simulink model "SensorlessBLDCMotorSimulation1"  (R2023a)
settings: Solver=VariableStepAuto  StartTime=0.0  StopTime=10.0  RelTol=1e-3
libraries: spsMosfetLib x6, spsPermanentMagnetSynchronousMachineLib x1, spsDCVoltageSourceLib x1, sps_lib x1
settings Model: Creator=ABRA A5 V16.6.1  LastModifiedBy=ABRA A5 V16.6.1

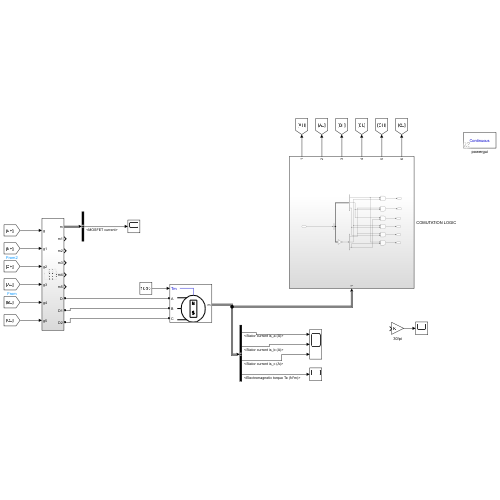
[thumbnail: Simulink's stored preview of the top-level diagram]
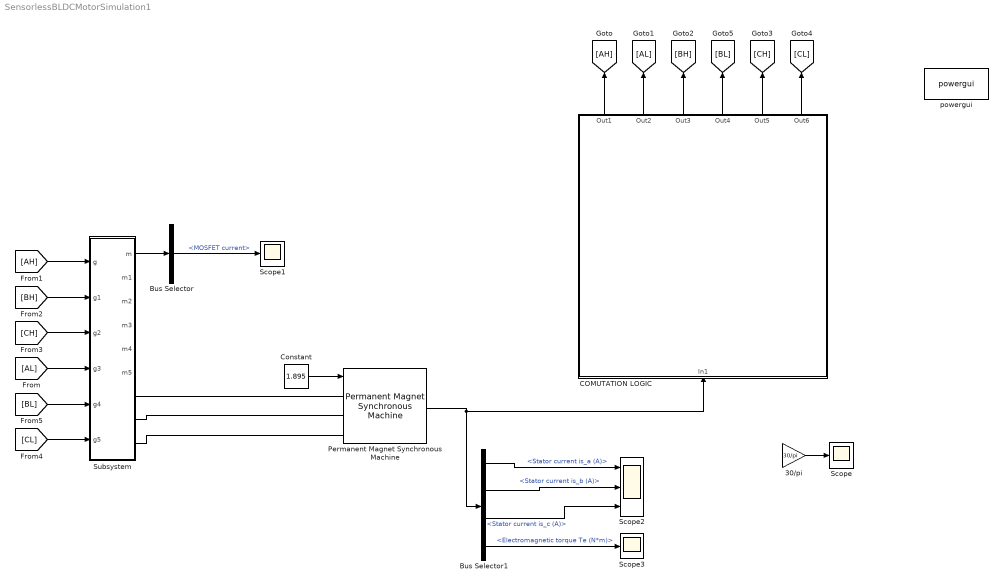
== system SensorlessBLDCMotorSimulation1 ==
  30/pi : Gain  Gain=30/pi
  Bus Selector : BusSelector  OutputSignals=MOSFET current
  Bus Selector1 : BusSelector  OutputSignals=Stator current is_a (A),Stator current is_b (A),Stator current is_c (A),Electromagnetic torque Te (N*m)
  COMUTATION LOGIC : Subsystem
  Constant : Constant  Value=1.895
  Permanent Magnet Synchronous Machine : spsPermanentMagnetSynchronousMachineLib/Permanent Magnet Synchronous Machine  NbPhases=3  FluxDistribution=Trapezoidal  RotorType=Round  MechanicalLoad=Torque Tm  PresetModel=No  ShowDetailedParameters=on  MeasurementBus=off  Resistance=0.0801  Inductance=0.0000841  dqInductances=[8.5e-3,8.5e-3]  La=0.000395  MachineConstant=Flux linkage established by magnets (V.s)  Flux=0.00216  VoltageCst=6.3335  TorqueCst=0.06048  Flat=120  Mechanical=[0.0002125 0.0004924 14 0]  PolePairs=4  InitialConditions=[314.159,-3.21, 30,30]  InitialConditions5ph=[0 0 0 0 0 0]  RefAngle=90 degrees behind phase A axis (modified Park)  IterativeDiscreteModel=Trapezoidal non iterative  TsBlock=-1  TsPowergui=0
  Scope : Scope
  Scope1 : Scope
  Scope2 : Scope  NumInputPorts=3
  Scope3 : Scope
  Subsystem : Subsystem
  powergui : sps_lib/powergui  Priority=1  SimulationMode=Continuous  SampleTime=50e-6  frequency=60  Iterations=50  frequencyindice=0  Pbase=100e6  ErrMax=1e-4  UnitsV=kV  UnitsW=MW  buscounter=0  FunctionMessages=off  echomessages=off  EnableUseOfTLC=off  CurrentSourceSwitches=off  DisableSnubberDevices=off  DisableRonSwitches=off  DisableVfSwitches=off  DisplayEquations=off  AutomaticDiscreteSolvers=off  SolverType=Tustin/Backward Euler (TBE)  Interpol=off  ExternalGateDelay=off  methode=off  Ts=100  x0status=blocks  SPID=on  SwTol=0  HookPort=off  NonlinearTolerance=1e-4  nMaxIteration=100  ContinueOnMaxIteration=off  RestoreLinks=warning  ResistiveCurrentMeasurement=off  Frange=[0:2:500]  Ylog=off  Xlog=on  ShowGrid=off  save=off  variable=ZData  structure=0  ZoomFFT=off  StartTime=0.0  cycles=1  DisplayStyle=1  fundamental=60  FreqAxis=off  MaxFrequency=1000  frequencyindicesteady=1  RmsSteady=1  display=off
  wires:
  Permanent Magnet Synchronous Machine/1 -> Bus Selector1/1, COMUTATION LOGIC/1(In1)
  COMUTATION LOGIC/1(Out1) -> [AH]
  COMUTATION LOGIC/2(Out2) -> [AL]
  COMUTATION LOGIC/3(Out3) -> [BH]
  COMUTATION LOGIC/4(Out4) -> [BL]
  COMUTATION LOGIC/5(Out5) -> [CH]
  COMUTATION LOGIC/6(Out6) -> [CL]
  [AH] -> Subsystem/1(g)
  [BH] -> Subsystem/2(g1)
  [CH] -> Subsystem/3(g2)
  [AL] -> Subsystem/4(g3)
  [BL] -> Subsystem/5(g4)
  [CL] -> Subsystem/6(g5)
  Subsystem/1(m) -> Bus Selector/1
  Bus Selector/1 -> Scope1/1  "<MOSFET current>"
  Constant/1 -> Permanent Magnet Synchronous Machine/1
  30/pi/1 -> Scope/1
  Bus Selector1/1 -> Scope2/1  "<Stator current is_a (A)>"
  Bus Selector1/2 -> Scope2/2  "<Stator current is_b (A)>"
  Bus Selector1/3 -> Scope2/3  "<Stator current is_c (A)>"
  Bus Selector1/4 -> Scope3/1  "<Electromagnetic torque Te (N*m)>"
  connections:
  Permanent Magnet Synchronous Machine/LConn1 -- Subsystem/RConn1
  Permanent Magnet Synchronous Machine/LConn2 -- Subsystem/RConn2
  Permanent Magnet Synchronous Machine/LConn3 -- Subsystem/RConn3

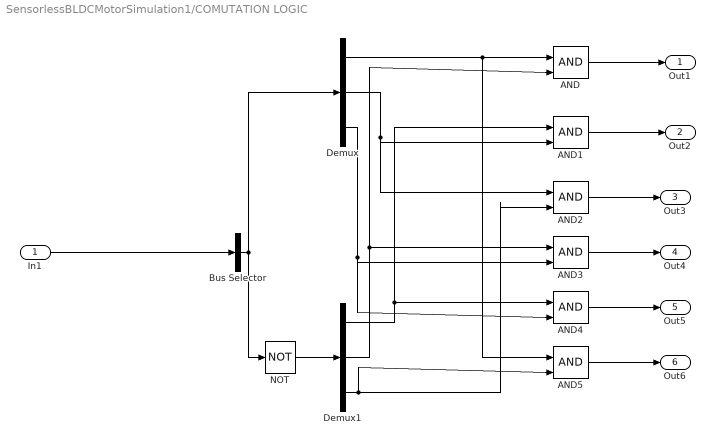
== system SensorlessBLDCMotorSimulation1/COMUTATION LOGIC ==
  In1 : Inport
  AND{,1..5} (6 alike) : Logic  IconShape=distinctive  AllPortsSameDT=off  OutDataTypeStr=boolean
  Bus Selector : BusSelector  OutputSignals=Hall effect signal h_a,Hall effect signal h_b,Hall effect signal h_c  OutputAsBus=on
  Demux : Demux  Outputs=3
  Demux1 : Demux  Outputs=3
  NOT : Logic  Operator=NOT  IconShape=distinctive  AllPortsSameDT=off  OutDataTypeStr=boolean
  Out1 : Outport
  Out2 : Outport  Port=2
  Out3 : Outport  Port=3
  Out4 : Outport  Port=4
  Out5 : Outport  Port=5
  Out6 : Outport  Port=6
  wires:
  AND3/1 -> Out4/1
  In1/1 -> Bus Selector/1
  Demux1/2 -> AND3/1, AND/2
  Bus Selector/1 -> Demux/1, NOT/1
  Demux/1 -> AND5/1, AND/1
  Demux/2 -> AND2/1, AND1/2
  Demux1/1 -> AND4/1, AND1/1
  AND4/1 -> Out5/1
  Demux1/3 -> AND5/2, AND2/2
  Demux/3 -> AND4/2, AND3/2
  AND2/1 -> Out3/1
  NOT/1 -> Demux1/1
  AND5/1 -> Out6/1
  AND/1 -> Out1/1
  AND1/1 -> Out2/1

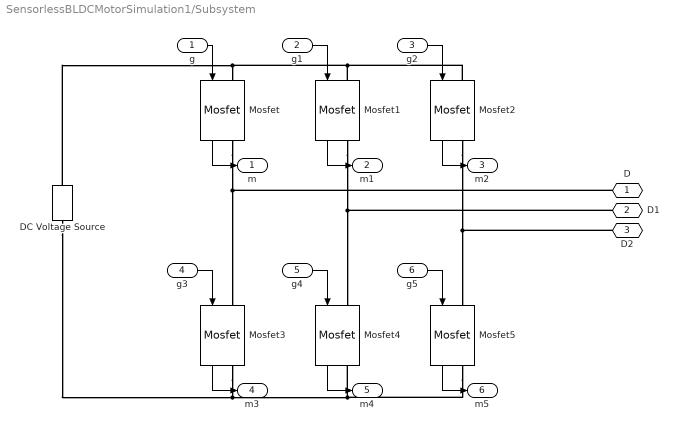
== system SensorlessBLDCMotorSimulation1/Subsystem ==
  g : Inport
  g1 : Inport  Port=2
  g2 : Inport  Port=3
  g3 : Inport  Port=4
  g4 : Inport  Port=5
  g5 : Inport  Port=6
  DC Voltage Source : spsDCVoltageSourceLib/DC Voltage Source  Amplitude=16.6  Measurements=Voltage
  Mosfet : spsMosfetLib/Mosfet  Ron=0.0175  Lon=0  Rd=0.0075  Vfd=1.33333  IC=0  Rs=1e5  Cs=inf  Measurements=on
  Mosfet{1..5} (5 alike) : spsMosfetLib/Mosfet  Ron=0.0175  Lon=0  Rd=0.0075  Vfd=1.3333  IC=0  Rs=1e5  Cs=inf  Measurements=on
  D : PMIOPort  Side=Right
  D1 : PMIOPort  Port=2  Side=Right
  D2 : PMIOPort  Port=3  Side=Right
  m : Outport
  m1 : Outport  Port=2
  m2 : Outport  Port=3
  m3 : Outport  Port=4
  m4 : Outport  Port=5
  m5 : Outport  Port=6
  wires:
  g5/1 -> Mosfet5/1
  Mosfet1/1 -> m1/1
  g3/1 -> Mosfet3/1
  Mosfet5/1 -> m5/1
  g1/1 -> Mosfet1/1
  g2/1 -> Mosfet2/1
  Mosfet3/1 -> m3/1
  g4/1 -> Mosfet4/1
  Mosfet4/1 -> m4/1
  Mosfet2/1 -> m2/1
  Mosfet/1 -> m/1
  g/1 -> Mosfet/1
  connections:
  Mosfet2/RConn1 -- D2/RConn1 -- Mosfet5/LConn1
  Mosfet1/LConn1 -- Mosfet2/LConn1 -- DC Voltage Source/RConn1 -- Mosfet/LConn1
  Mosfet3/RConn1 -- DC Voltage Source/LConn1 -- Mosfet5/RConn1 -- Mosfet4/RConn1
  Mosfet1/RConn1 -- D1/RConn1 -- Mosfet4/LConn1
  Mosfet/RConn1 -- D/RConn1 -- Mosfet3/LConn1
